simulink model "s_tanks_1"  (Simulink 10.3)
settings: Solver=ode4  StartTime=0.0  StopTime=60  FixedStep=0.002  RelTol=1e-3  EnableMultiTasking=on
undefined symbols (not defined in the file or in its folder): Ao1, At1, g, Kff_1, Ki_1, Kp, Kp_1, L10, MAX_L1_WDUP, TS, VMAX_AMP
settings Model: Creator=MLevis  LastModifiedBy=tronc  ExtModeTrigDuration=30000
settings SolverCC: PositivePriorityOrder=on
settings DataIOCC: LimitDataPoints=on
settings OptimizationCC: InitFltsAndDblsToZero=on
settings DebuggingCC: SaveWithParameterizedLinksMsg=none  SolverPrmCheckMsg=warning
settings SFSimCC: SimUseLocalCustomCode=on  CustomCodeUndefinedFunction=FilterOut
settings RTWCC: Description=QuaRC Win32 Target  SystemTargetFile=quarc_windows.tlc  TemplateMakefile=quarc_default_tmf  RTWUseLocalCustomCode=on
settings STFCustomTargetCC: TargetFcnLib=ansi_tfl_tmw.mat  TargetPreCompLibLocation=C:\DOCUME~1\ALLUSE~1\APPLIC~1\QUARC\lib\2007b\windows\release  CPPClassGenCompliant=on  SystemTargetFile=quarc_windows.tlc
settings GRTTargetCC: TargetFcnLib=ansi_tfl_tmw.mat  TargetPreCompLibLocation=C:\DOCUME~1\ALLUSE~1\APPLIC~1\QUARC\lib\2007b\windows\release  ParMdlRefBuildCompliant=off  CompOptLevelCompliant=off  ConcurrentExecutionCompliant=off  MatFileLogging=off  UseToolchainInfoCompliant=off  ExtMode=on  ExtModeMexFile=quarc_comm
settings ConfigComp: CovExternalEMLEnable=on

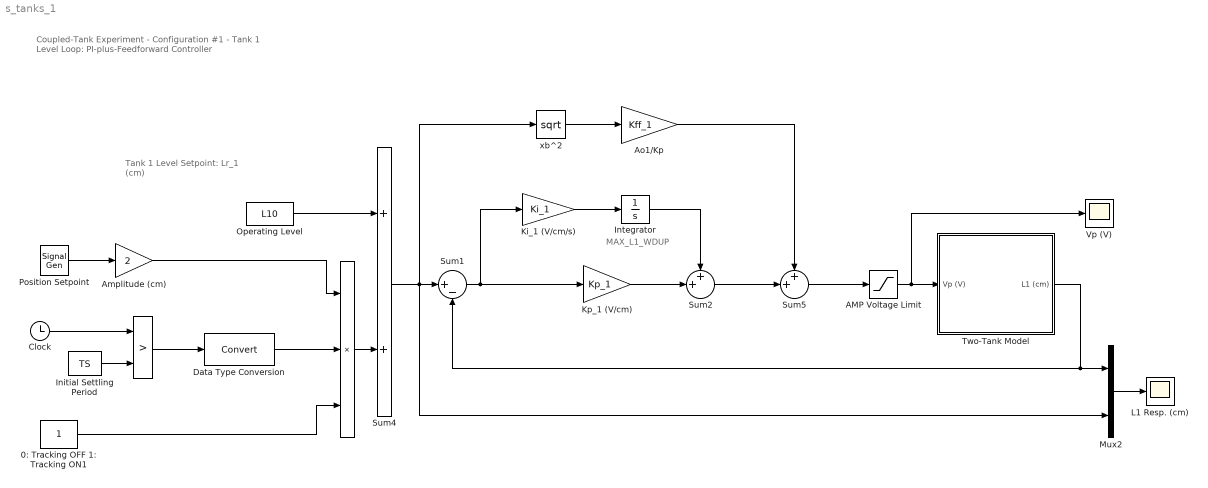
== system s_tanks_1 ==
  note: Coupled-Tank Experiment
      | - Configuration #1 -
      | Tank 1 Level Loop:
      | PI-plus-Feedforward Controller
  note: Tank 1 Level Setpoint:
      | Lr_1 (cm)
  note: MAX_L1_WDUP
  "   " : Product  Inputs=3  InputSameDT=on  RndMeth=Zero  SaturateOnIntegerOverflow=on  OutDataTypeStr=Inherit: Same as first input
  "    " : RelationalOperator  Operator=>  RndMeth=Nearest  InputSameDT=on
  0: Tracking OFF 1: Tracking ON1 : Constant
  AMP Voltage Limit : Saturate  UpperLimit=VMAX_AMP  LowerLimit=0
  Amplitude (cm) : Gain  Gain=2  SaturateOnIntegerOverflow=on  OutDataTypeStr=Inherit: Same as input  ParamDataTypeStr=Inherit: Same as input
  Ao1/Kp : Gain  Gain=Kff_1  SaturateOnIntegerOverflow=on  OutDataTypeStr=Inherit: Same as input  ParamDataTypeStr=Inherit: Same as input
  Clock : Clock
  Data Type Conversion : DataTypeConversion
  Initial Settling Period : Constant  Value=TS
  Integrator : Integrator  LimitOutput=on  UpperSaturationLimit=MAX_L1_WDUP  LowerSaturationLimit=- MAX_L1_WDUP
  Ki_1 (V/cm/s) : Gain  Gain=Ki_1  SaturateOnIntegerOverflow=on  OutDataTypeStr=Inherit: Same as input  ParamDataTypeStr=Inherit: Same as input
  Kp_1 (V/cm) : Gain  Gain=Kp_1  SaturateOnIntegerOverflow=on  OutDataTypeStr=Inherit: Same as input  ParamDataTypeStr=Inherit: Same as input
  L1 Resp. (cm) : Scope
  Mux2 : Mux  Inputs=2
  Operating Level : Constant  Value=L10
  Position Setpoint : SignalGenerator  WaveForm=square  Frequency=0.05
  Sum1 : Sum  Inputs=|+-  InputSameDT=on  SaturateOnIntegerOverflow=on  OutDataTypeStr=Inherit: Same as first input
  Sum2 : Sum  Inputs=++|  InputSameDT=on  SaturateOnIntegerOverflow=on  OutDataTypeStr=Inherit: Same as first input
  Sum4 : Sum  InputSameDT=on  SaturateOnIntegerOverflow=on  OutDataTypeStr=Inherit: Same as first input
  Sum5 : Sum  Inputs=++|  InputSameDT=on  SaturateOnIntegerOverflow=on  OutDataTypeStr=Inherit: Same as first input
  Two-Tank Model : Subsystem
  "Vp (V) " : Scope
  xb^2 : Math  Operator=sqrt  SignedPower=on  SaturateOnIntegerOverflow=on
  wires:
  Mux2/1 -> L1 Resp. (cm)/1
  Sum1/1 -> Kp_1 (V/cm)/1, Ki_1 (V/cm/s)/1
  Ki_1 (V/cm/s)/1 -> Integrator/1
  Kp_1 (V/cm)/1 -> Sum2/2
  Integrator/1 -> Sum2/1
  AMP Voltage Limit/1 -> Two-Tank Model/1(Vp (V)), "Vp (V) "/1
  Sum4/1 -> xb^2/1, Sum1/1, Mux2/2
  Sum2/1 -> Sum5/2
  Sum5/1 -> AMP Voltage Limit/1
  xb^2/1 -> Ao1/Kp/1
  Ao1/Kp/1 -> Sum5/1
  Two-Tank Model/1(L1 (cm)) -> Sum1/2, Mux2/1
  Position Setpoint/1 -> Amplitude (cm)/1
  0: Tracking OFF 1: Tracking ON1/1 -> "   "/3
  "   "/1 -> Sum4/2
  Operating Level/1 -> Sum4/1
  Initial Settling Period/1 -> "    "/2
  Clock/1 -> "    "/1
  Amplitude (cm)/1 -> "   "/1
  "    "/1 -> Data Type Conversion/1
  Data Type Conversion/1 -> "   "/2

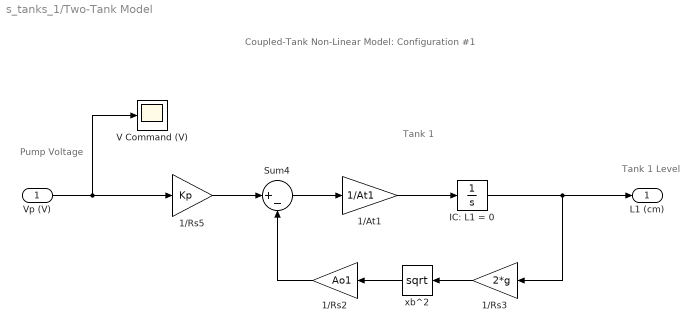
== system s_tanks_1/Two-Tank Model ==
  note: Coupled-Tank Non-Linear Model:
      | Configuration #1
  note: Tank 1
  note: Tank 1 Level
  note: Pump
      | Voltage
  Vp (V) : Inport
  1/At1 : Gain  Gain=1/At1  SaturateOnIntegerOverflow=on  OutDataTypeStr=Inherit: Same as input  ParamDataTypeStr=Inherit: Same as input
  1/Rs2 : Gain  Gain=Ao1  SaturateOnIntegerOverflow=on  OutDataTypeStr=Inherit: Same as input  ParamDataTypeStr=Inherit: Same as input
  1/Rs3 : Gain  Gain=2*g  SaturateOnIntegerOverflow=on  OutDataTypeStr=Inherit: Same as input  ParamDataTypeStr=Inherit: Same as input
  1/Rs5 : Gain  Gain=Kp  SaturateOnIntegerOverflow=on  OutDataTypeStr=Inherit: Same as input  ParamDataTypeStr=Inherit: Same as input
  IC: L1 = 0 : Integrator
  Sum4 : Sum  Inputs=|+-  InputSameDT=on  SaturateOnIntegerOverflow=on  OutDataTypeStr=Inherit: Same as first input
  V Command (V) : Scope
  xb^2 : Math  Operator=sqrt  SignedPower=on  SaturateOnIntegerOverflow=on
  L1 (cm) : Outport  InitialOutput=0
  wires:
  Vp (V)/1 -> V Command (V)/1, 1/Rs5/1
  1/Rs5/1 -> Sum4/1
  Sum4/1 -> 1/At1/1
  1/At1/1 -> IC: L1 = 0/1
  IC: L1 = 0/1 -> 1/Rs3/1, L1 (cm)/1
  1/Rs2/1 -> Sum4/2
  xb^2/1 -> 1/Rs2/1
  1/Rs3/1 -> xb^2/1
